simulink model "s_hover"  (Simulink 8.8)
settings: Solver=ode14x  StartTime=0.0  StopTime=inf  FixedStep=0.005  RelTol=1e-3  EnableMultiTasking=on
values from neighbouring files (symbols this model uses):
  CMD_RATE_LIMIT = 60 * pi/180    (= 1.0471975512)    [Copy_of_setup_lab_hover.m]    (also in setup_lab_hover.m; setup_lab_hover1.m)
  K = lqr( A, B, Q, R )    [setup_lab_hover.m]    (also in setup_lab_hover1.m)
  K_AMP = 3    [Copy_of_setup_lab_hover.m]    (also in setup_lab_hover.m; setup_lab_hover1.m)
  V_bias = 2.0    (= 2)    [setup_lab_hover.m]    (also in setup_lab_hover1.m)
  VMAX_AMP = 24    [Copy_of_setup_lab_hover.m]    (also in setup_lab_hover.m; setup_lab_hover1.m)
  VMAX_DAC = 10    [Copy_of_setup_lab_hover.m]    (also in setup_lab_hover.m; setup_lab_hover1.m)
  wcf = 2 * pi * 20    (= 125.663706144)    [Copy_of_setup_lab_hover.m]    (also in setup_lab_hover.m; setup_lab_hover1.m)
  zetaf = 0.6    [Copy_of_setup_lab_hover.m]    (also in setup_lab_hover.m; setup_lab_hover1.m)
undefined symbols (not defined in the file or in its folder): A, B, C, D
libraries: simulink_extras x5, instrumentlib x2, aerolibanimutils x1
settings Model: SuppressorTable=22 serialization::archive 11 0 3 0 0 0 0 0  Creator=hpineros  LastModifiedBy=ronan  ExtModeTrigDuration=10000
settings SolverCC: PositivePriorityOrder=on
settings OptimizationCC: ExpressionDepthLimit=2147483647  InitFltsAndDblsToZero=on
settings DebuggingCC: SaveWithParameterizedLinksMsg=none  SolverPrmCheckMsg=warning
settings RTWCC: SystemTargetFile=quarc_windows.tlc  TemplateMakefile=quarc_default_tmf  Description=QuaRC Win32 Target
settings STFCustomTargetCC: TargetFcnLib=ansi_tfl_tmw.mat  TargetPreCompLibLocation=C:\PROGRA~3\QUARC\lib\2012b\windows\release  GeneratePreprocessorConditionals=Disable all  CPPClassGenCompliant=on  SystemTargetFile=quarc_windows.tlc
settings GRTTargetCC: TargetFcnLib=ansi_tfl_tmw.mat  TargetPreCompLibLocation=C:\PROGRA~3\QUARC\lib\2012b\windows\release  ParMdlRefBuildCompliant=off  CompOptLevelCompliant=off  ConcurrentExecutionCompliant=off  MatFileLogging=off  UseToolchainInfoCompliant=off  ExtMode=on  ExtModeMexFile=quarc_comm

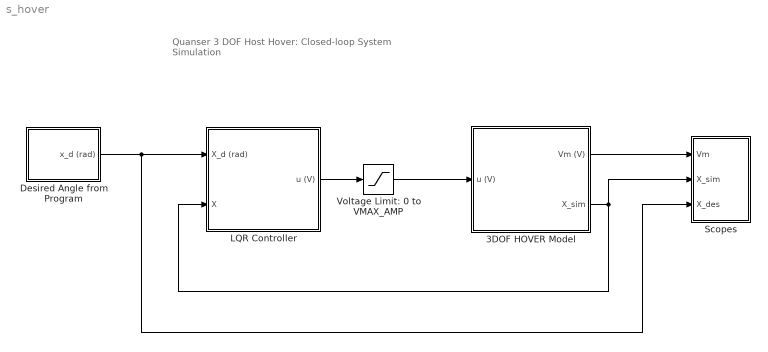
== system s_hover ==
  note: Quanser 3 DOF Host Hover:
      | Closed-loop System Simulation
  3DOF HOVER Model : Subsystem
  Desired Angle from Program : Subsystem
  LQR Controller : Subsystem
  Scopes : Subsystem
  Voltage Limit: 0 to VMAX_AMP : Saturate  UpperLimit=VMAX_AMP  LowerLimit=0
  wires:
  Desired Angle from Program/1(x_d (rad)) -> LQR Controller/1(X_d (rad)), Scopes/3(X_des)
  Voltage Limit: 0 to VMAX_AMP/1 -> 3DOF HOVER Model/1(u (V))
  3DOF HOVER Model/1(Vm (V)) -> Scopes/1(Vm)
  LQR Controller/1(u (V)) -> Voltage Limit: 0 to VMAX_AMP/1
  3DOF HOVER Model/2(X_sim) -> LQR Controller/2(X), Scopes/2(X_sim)

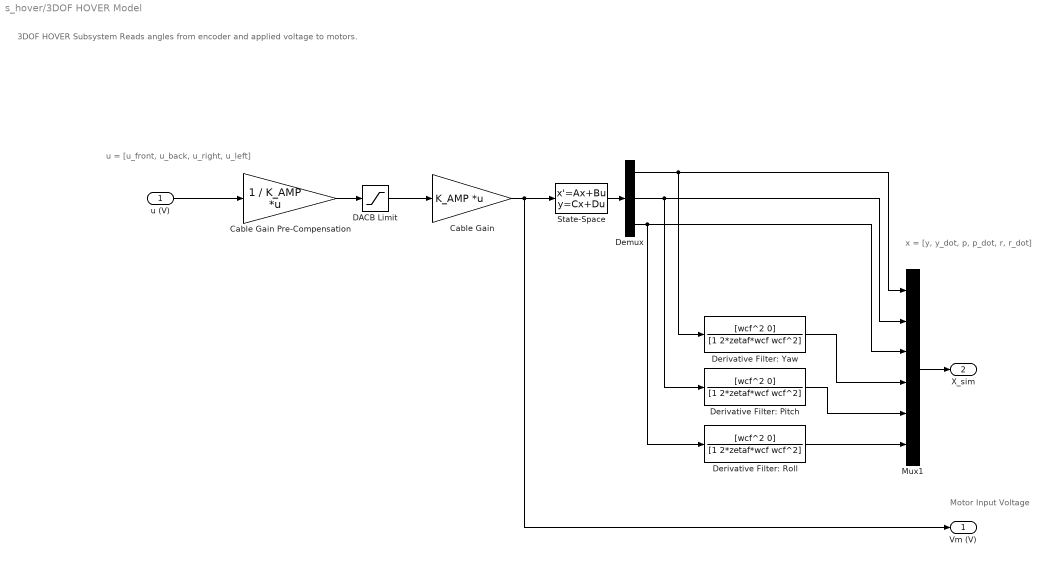
== system s_hover/3DOF HOVER Model ==
  note: 3DOF HOVER Subsystem
      | Reads angles from encoder and applied voltage to motors.
  note: Motor Input Voltage
  note: u = [u_front, u_back, u_right, u_left]
  note: x = [y, y_dot, p, p_dot, r, r_dot]
  u (V) : Inport
  Cable Gain : Gain  Gain=K_AMP  Multiplication=Matrix(K*u)  SaturateOnIntegerOverflow=on  OutDataTypeStr=Inherit: Same as input  ParamDataTypeStr=Inherit: Same as input
  Cable Gain Pre-Compensation : Gain  Gain=1 / K_AMP  Multiplication=Matrix(K*u)  SaturateOnIntegerOverflow=on  OutDataTypeStr=Inherit: Same as input  ParamDataTypeStr=Inherit: Same as input
  DACB Limit : Saturate  UpperLimit=VMAX_DAC  LowerLimit=-VMAX_DAC
  Demux : Demux  Outputs=3
  Derivative Filter: Pitch : TransferFcn  Numerator=[wcf^2 0]  Denominator=[1 2*zetaf*wcf wcf^2]
  Derivative Filter: Roll : TransferFcn  Numerator=[wcf^2 0]  Denominator=[1 2*zetaf*wcf wcf^2]
  Derivative Filter: Yaw : TransferFcn  Numerator=[wcf^2 0]  Denominator=[1 2*zetaf*wcf wcf^2]
  Mux1 : Mux  Inputs=6
  State-Space : StateSpace  A=A  B=B  C=C  D=D  X0=0
  Vm (V) : Outport
  X_sim : Outport  Port=2
  wires:
  Demux/3 -> Derivative Filter: Roll/1, Mux1/3
  Demux/2 -> Derivative Filter: Pitch/1, Mux1/2
  Derivative Filter: Roll/1 -> Mux1/6
  Derivative Filter: Pitch/1 -> Mux1/5
  Derivative Filter: Yaw/1 -> Mux1/4
  Demux/1 -> Derivative Filter: Yaw/1, Mux1/1
  State-Space/1 -> Demux/1
  Mux1/1 -> X_sim/1
  Cable Gain/1 -> State-Space/1, Vm (V)/1
  DACB Limit/1 -> Cable Gain/1
  Cable Gain Pre-Compensation/1 -> DACB Limit/1
  u (V)/1 -> Cable Gain Pre-Compensation/1

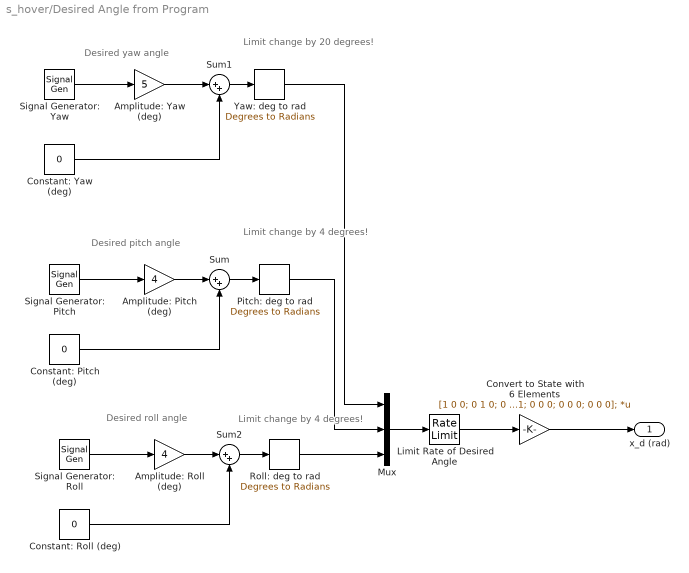
== system s_hover/Desired Angle from Program ==
  note: Limit change by
      | 4 degrees!
  note: Limit change by
      | 20 degrees!
  note: Limit change by
      | 4 degrees!
  note: Desired roll angle
  note: Desired pitch angle
  note: Desired yaw angle
  Amplitude: Pitch (deg) : Gain  Gain=4
  Amplitude: Roll (deg) : Gain  Gain=4
  Amplitude: Yaw (deg) : Gain  Gain=5
  Constant: Pitch (deg) : Constant  Value=0
  Constant: Roll (deg) : Constant  Value=0
  Constant: Yaw (deg) : Constant  Value=0
  Convert to State with 6 Elements : Gain  Gain=[1 0 0; 0 1 0; 0 0 1; 0 0 0; 0 0 0; 0 0 0];  Multiplication=Matrix(K*u)
  Limit Rate of Desired Angle : RateLimiter  RisingSlewLimit=CMD_RATE_LIMIT  FallingSlewLimit=-CMD_RATE_LIMIT
  Mux : Mux  Inputs=3
  Pitch: deg to rad : simulink_extras/Transformations/Degrees to Radians
  Roll: deg to rad : simulink_extras/Transformations/Degrees to Radians
  Signal Generator: Pitch : SignalGenerator  WaveForm=square  Frequency=0.1
  Signal Generator: Roll : SignalGenerator  WaveForm=square  Frequency=0.08
  Signal Generator: Yaw : SignalGenerator  WaveForm=square  Frequency=0.04
  Sum : Sum  Inputs=|++
  Sum1 : Sum  Inputs=|++
  Sum2 : Sum  Inputs=|++
  Yaw: deg to rad : simulink_extras/Transformations/Degrees to Radians
  x_d (rad) : Outport
  wires:
  Convert to State with 6 Elements/1 -> x_d (rad)/1
  Limit Rate of Desired Angle/1 -> Convert to State with 6 Elements/1
  Roll: deg to rad/1 -> Mux/3
  Pitch: deg to rad/1 -> Mux/2
  Yaw: deg to rad/1 -> Mux/1
  Sum2/1 -> Roll: deg to rad/1
  Signal Generator: Roll/1 -> Amplitude: Roll (deg)/1
  Amplitude: Roll (deg)/1 -> Sum2/1
  Constant: Roll (deg)/1 -> Sum2/2
  Sum/1 -> Pitch: deg to rad/1
  Signal Generator: Pitch/1 -> Amplitude: Pitch (deg)/1
  Amplitude: Pitch (deg)/1 -> Sum/1
  Constant: Pitch (deg)/1 -> Sum/2
  Sum1/1 -> Yaw: deg to rad/1
  Signal Generator: Yaw/1 -> Amplitude: Yaw (deg)/1
  Amplitude: Yaw (deg)/1 -> Sum1/1
  Constant: Yaw (deg)/1 -> Sum1/2
  Mux/1 -> Limit Rate of Desired Angle/1

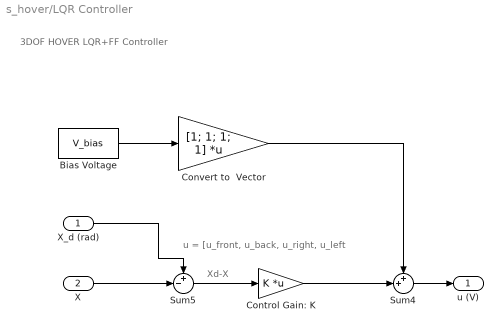
== system s_hover/LQR Controller ==
  note: u = [u_front, u_back, u_right, u_left
  note: Xd-X
  note: 3DOF HOVER LQR+FF Controller
  X_d (rad) : Inport
  X : Inport  Port=2
  Bias Voltage : Constant  Value=V_bias
  Control Gain: K : Gain  Gain=K  Multiplication=Matrix(K*u)
  Convert to  Vector : Gain  Gain=[1; 1; 1; 1]  Multiplication=Matrix(K*u)
  Sum4 : Sum  Inputs=++|
  Sum5 : Sum  Inputs=+-|
  u (V) : Outport
  wires:
  Sum5/1 -> Control Gain: K/1
  X/1 -> Sum5/2
  X_d (rad)/1 -> Sum5/1
  Convert to  Vector/1 -> Sum4/1
  Control Gain: K/1 -> Sum4/2
  Bias Voltage/1 -> Convert to  Vector/1
  Sum4/1 -> u (V)/1

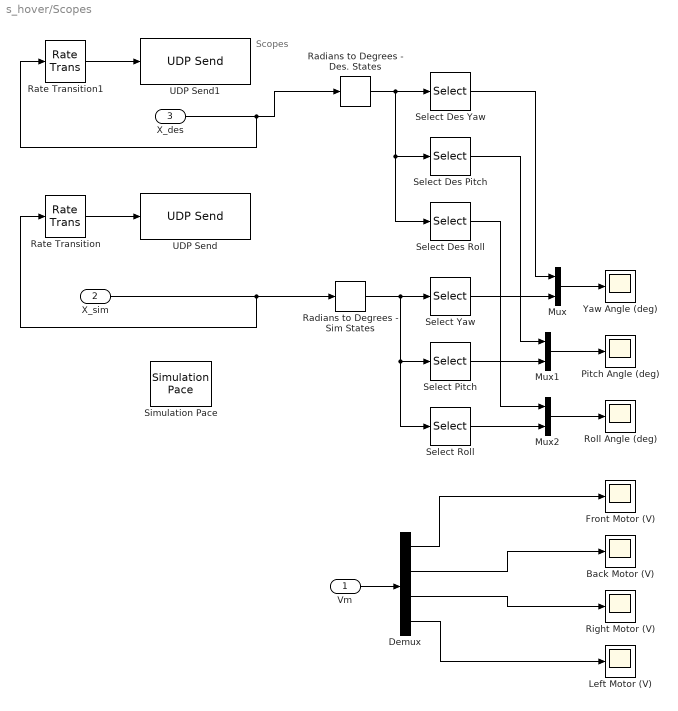
== system s_hover/Scopes ==
  note: Scopes
  Vm : Inport
  X_sim : Inport  Port=2
  X_des : Inport  Port=3
  Back Motor (V) : Scope
  Demux : Demux
  Front Motor (V) : Scope
  Left Motor (V) : Scope
  Mux : Mux  Inputs=2
  Mux1 : Mux  Inputs=2
  Mux2 : Mux  Inputs=2
  Pitch Angle (deg) : Scope
  Radians to Degrees - Des. States : simulink_extras/Transformations/Radians to Degrees
  Radians to Degrees - Sim States : simulink_extras/Transformations/Radians to Degrees
  Rate Transition : RateTransition  OutPortSampleTime=0.005
  Rate Transition1 : RateTransition  OutPortSampleTime=0.005
  Right Motor (V) : Scope
  Roll Angle (deg) : Scope
  Select Des Pitch : Selector  InputPortWidth=6  IndexOptions=Index vector (dialog)  Indices=2  OutputSizes=1
  Select Des Roll : Selector  InputPortWidth=6  IndexOptions=Index vector (dialog)  Indices=3  OutputSizes=1
  Select Des Yaw : Selector  InputPortWidth=6  IndexOptions=Index vector (dialog)  Indices=1  OutputSizes=1
  Select Pitch : Selector  InputPortWidth=6  IndexOptions=Index vector (dialog)  Indices=2  OutputSizes=1
  Select Roll : Selector  InputPortWidth=6  IndexOptions=Index vector (dialog)  Indices=3  OutputSizes=1
  Select Yaw : Selector  InputPortWidth=6  IndexOptions=Index vector (dialog)  Indices=1  OutputSizes=1
  Simulation Pace : aerolibanimutils/Simulation Pace  SimulationPace=1  SleepMode=MATLAB Thread  OutputPaceError=off  SampleTime=0.01
  UDP Send : instrumentlib/UDP Send  Host=localhost  Port=9092  LocalPort=9091  EnableBlockingMode=on  ByteOrder=BigEndian
  UDP Send1 : instrumentlib/UDP Send  Host=localhost  Port=9094  LocalPort=9093  EnableBlockingMode=on  ByteOrder=BigEndian
  Yaw Angle (deg) : Scope
  wires:
  Select Des Roll/1 -> Mux2/1
  Select Des Pitch/1 -> Mux1/1
  Select Des Yaw/1 -> Mux/1
  Radians to Degrees - Des. States/1 -> Select Des Roll/1, Select Des Pitch/1, Select Des Yaw/1
  Select Roll/1 -> Mux2/2
  Select Pitch/1 -> Mux1/2
  Select Yaw/1 -> Mux/2
  Mux2/1 -> Roll Angle (deg)/1
  Radians to Degrees - Sim States/1 -> Select Roll/1, Select Pitch/1, Select Yaw/1
  Mux1/1 -> Pitch Angle (deg)/1
  Mux/1 -> Yaw Angle (deg)/1
  X_sim/1 -> Radians to Degrees - Sim States/1, Rate Transition/1
  Vm/1 -> Demux/1
  Demux/1 -> Front Motor (V)/1
  Demux/2 -> Back Motor (V)/1
  Demux/3 -> Right Motor (V)/1
  Demux/4 -> Left Motor (V)/1
  Rate Transition/1 -> UDP Send/1
  X_des/1 -> Rate Transition1/1, Radians to Degrees - Des. States/1
  Rate Transition1/1 -> UDP Send1/1
